simulink model "method2"  (R2025a)
settings: Solver=ode45  StartTime=0.0  StopTime=100  MaxStep=0.01  RelTol=1e-3
settings Model: Creator=vm66c  LastModifiedBy=vm66c

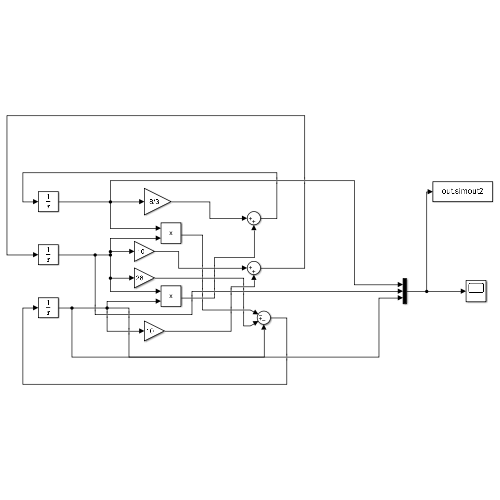
[thumbnail: Simulink's stored preview of the top-level diagram]
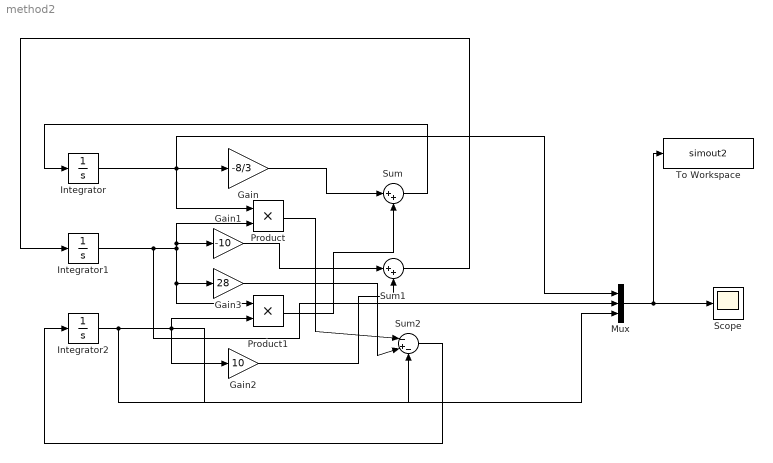
== system method2 ==
  Gain : Gain  Gain=-8/3
  Gain1 : Gain  Gain=-10
  Gain2 : Gain  Gain=10
  Gain3 : Gain  Gain=28
  Integrator : Integrator
  Integrator1 : Integrator
  Integrator2 : Integrator  InitialCondition=1e-10
  Mux : Mux  Inputs=3
  Product : Product
  Product1 : Product
  Scope : Scope
      settings: ActiveDisplayYMinimum=-41.040602957052272  ActiveDisplayYMaximum=59.321150562625462
  Sum : Sum  Inputs=|++
  Sum1 : Sum  Inputs=|++
  Sum2 : Sum  Inputs=|-+-
  To Workspace : ToWorkspace  VariableName=simout2  SampleTime=-1
  wires:
  Integrator/1 -> Mux/1, Gain/1, Product/1
  Integrator1/1 -> Mux/2, Gain1/1, Product/2, Gain3/1, Product1/1
  Integrator2/1 -> Mux/3, Sum2/3, Product1/2, Gain2/1
  Gain/1 -> Sum/1
  Product1/1 -> Sum/2
  Gain1/1 -> Sum1/1
  Gain2/1 -> Sum1/2
  Product/1 -> Sum2/1
  Gain3/1 -> Sum2/2
  Sum/1 -> Integrator/1
  Sum1/1 -> Integrator1/1
  Sum2/1 -> Integrator2/1
  Mux/1 -> To Workspace/1, Scope/1
